simulink model "ex3_sim"  (R2020b)
settings: Solver=VariableStepAuto  StartTime=0.0  StopTime=10.0  RelTol=1e-3
undefined symbols (not defined in the file): A, B, C, K, N
settings Model: Creator=ldrag  LastModifiedBy=ldrag

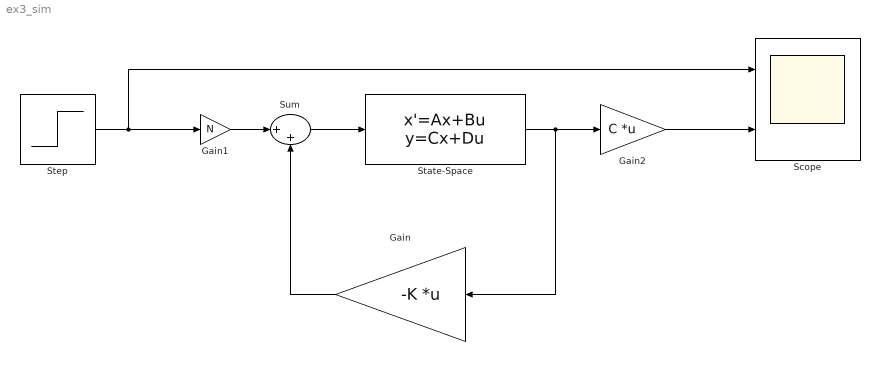
== system ex3_sim ==
  Gain : Gain  Gain=-K  Multiplication=Matrix(K*u) (u vector)
  Gain1 : Gain  Gain=N
  Gain2 : Gain  Gain=C  Multiplication=Matrix(K*u) (u vector)
  Scope : Scope  NumInputPorts=2
  State-Space : StateSpace  A=A  B=B  C=eye(3)  D=[0;0;0]  InitialCondition=0
  Step : Step  SampleTime=0
  Sum : Sum  Inputs=|++
  wires:
  Step/1 -> Scope/1, Gain1/1
  Sum/1 -> State-Space/1
  Gain1/1 -> Sum/1
  Gain2/1 -> Scope/2
  Gain/1 -> Sum/2
  State-Space/1 -> Gain/1, Gain2/1
